simulink model "microNole_MPC2021"  (R2022b)
settings: Solver=VariableStepAuto  StartTime=0.0  StopTime=100  RelTol=1e-3
values from neighbouring files (symbols this model uses):
  Theta3 = Theta{1,3}    [MicroNole_dynamics.m]
  Theta4 = Theta{1,4}    [MicroNole_dynamics.m]
  Theta5 = Theta{1,5}    [MicroNole_dynamics.m]
  Theta6 = Theta3*Theta5/Theta4    [MicroNole_dynamics.m]
undefined symbols (not defined in the file or in its folder): b1, b2, b_bar, d0, desired_longitudinal_speed, double_lane_flag, F1, F2, h, H1, H2, H_bar, K1, K_mpc_clock, K_mpc_counterclock, Ki1, Kp1, L, M, n_input, n_states, omegam0, p1, p2, rg, Rw, sat_pwm, sat_steering, Theta1, Theta2, Ts, V0, X0, x_boundary
settings Model: Creator=zysgh  LastModifiedBy=Abelb
settings DebuggingCC: UnconnectedInputMsg=warning  UnconnectedOutputMsg=warning  UnconnectedLineMsg=warning
settings ModelReferenceCC: EnableRefExpFcnMdlSchedulingChecks=on
settings RTWCC: DLArmComputeVersion=19.05

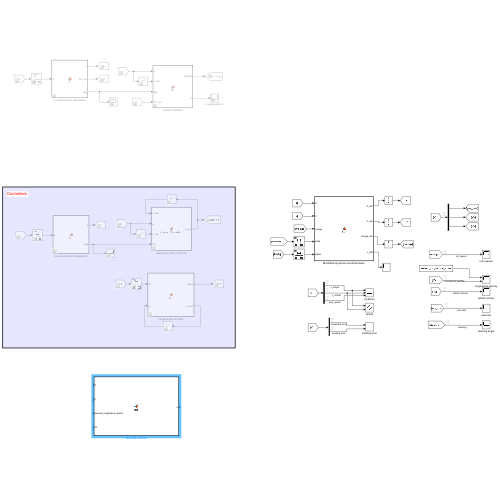
[thumbnail: Simulink's stored preview of the top-level diagram]
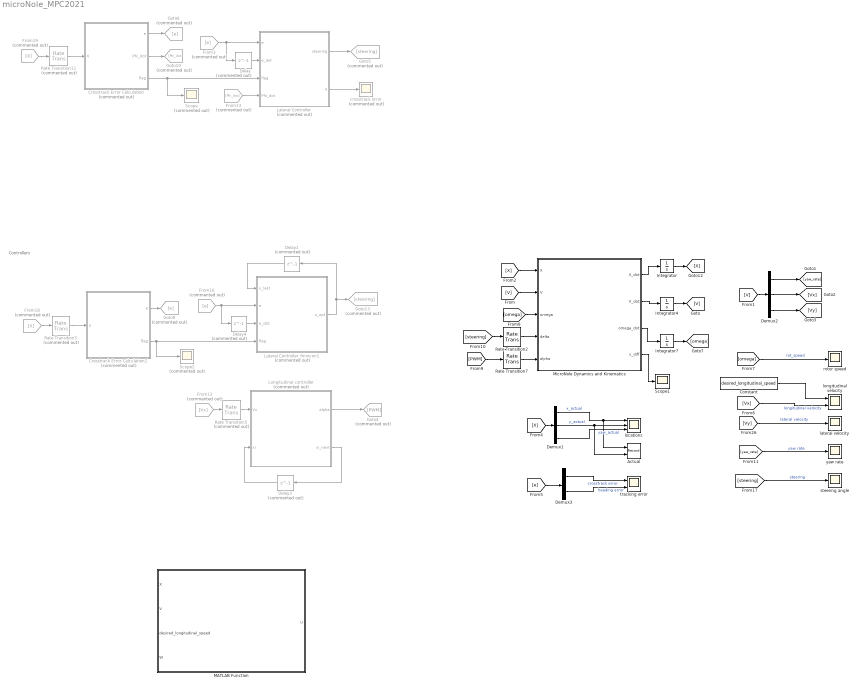
== system microNole_MPC2021 ==
  note: Controllers
  Actual : Record  FileSettingsInternal="{\"entries\":[{\"content\":{\"excelSettings\":{\"content\":{},\"type\":\"Streamout.ExcelSettings\"}},\"type\":\"Streamout.FileSettingStorage\",\"uuid\":\"74785e19-3353-448a-b1e4-8c9a9f0e60d2\"}],\"packageUris\":[\"http://schema.mathworks.com/mf0/streamout_blocks/R2020a\"],\"version\":\"1.0\"}"  Layout=[1 1]  SignalsInternal="{\"entries\":[{\"content\":{\"signals\":[{\"content\":{\"blockPath\":[\"microNole_MPC2021/Actual\"],\"channel\":[],\"dimensions\":[1],\"domain\":\"microNole_MPC2021/Actual\",\"lineColor\":\"#a2142f\",\"plots\":[1],\"port\":1,\"sid\":[\"\"],\"signalID\":1557,\"signalName\":\"x_actual\"},\"type\":\"RecordBlkView.Signal\",\"uuid\":\"f191aebf-62f9-445e-8cf5-1f0d9c420840\"},{\"content\":{\"blockPath\":[\"microNole_MPC2021/Actual\"],\"channel\":[],\"dimensions\":[1],\"domain\":\"microNole_MPC2021/Actual\",\"lineColor\":\"#139fff\",\"plots\":[1],\"port\":2,\"sid\":[\"\"],\"signalID\":1561,\"signalName\":\"y_actual\"},\"type\":\"RecordBlkView.Signal\",\"uuid\":\"59f82387-b242-4805-80ba-ae25613a261f\"}]},\"type\":\"RecordBlkView.InputSignals\",\"uuid\":\"e4cdd9aa-afbb-4b03-ab14-af52f1503f9a\"}],\"packageUris\":[\"http://schema.mathworks.com/mf0/streamout_blocks/R2020a\"],\"version\":\"1.0\"}"  VisualizationBindings="{\"xyplotplugin\":{\"info\":[{\"series\":[{\"bindingParametersList\":[{\"parameter\":\"X-Axis\",\"signalID\":1557,\"signalName\":\"x_actual\"},{\"parameter\":\"Y-Axis\",\"signalID\":1561,\"signalName\":\"y_actual\"}],\"seriesID\":12829}],\"subplotID\":1}]}}"  CompatibilityTag=XY  st=-1
  Constant : Constant  Value=desired_longitudinal_speed
  Crosstrack Error Calculation : MATLAB Function  Commented=on  TreatAsAtomicUnit=on
  Crosstrack Error Calculation2 : MATLAB Function  Commented=on  TreatAsAtomicUnit=on
  Delay : Delay  Commented=on  DelayLength=1  InitialCondition=[e10; e20]  SampleTime=Ts
  Delay1 : Delay  Commented=on  DelayLength=1  SampleTime=Ts
  Delay3 : Delay  Commented=on  DelayLength=1  SampleTime=Ts
  Delay4 : Delay  Commented=on  DelayLength=1  InitialCondition=[e10; e20]  SampleTime=Ts
  Demux1 : Demux  Outputs=3
  Demux2 : Demux  Outputs=3
  Demux3 : Demux  Outputs=2
  From12 : From  Commented=on  GotoTag=Vx
  From13 : From  Commented=on  GotoTag=Phi_dot
  From16 : From  Commented=on  GotoTag=e
  From18 : From  Commented=on  GotoTag=X
  From19 : From  Commented=on  GotoTag=X
  From3 : From  Commented=on  GotoTag=e
  Goto10 : Goto  Commented=on  GotoTag=Phi_dot
  Goto13 : Goto  Commented=on  GotoTag=steering
  Goto4 : Goto  Commented=on  GotoTag=PWM
  Goto5 : Goto  Commented=on  GotoTag=steering
  Goto6 : Goto  Commented=on  GotoTag=e
  Goto9 : Goto  Commented=on  GotoTag=e
  Integrator : Integrator  InitialCondition=X0
  Integrator4 : Integrator  InitialCondition=V0
  Integrator7 : Integrator  InitialCondition=omegam0
  Lateral Controller : MATLAB Function  Commented=on  TreatAsAtomicUnit=on
  Lateral Controller_fmincon1 : MATLAB Function  Commented=on  TreatAsAtomicUnit=on
  Longitudinal controller : MATLAB Function  Commented=on  TreatAsAtomicUnit=on
  MATLAB Function : MATLAB Function  TreatAsAtomicUnit=on
  MicroNole Dynamics and Kinematics : MATLAB Function  TreatAsAtomicUnit=on
  Rate Transition11 : RateTransition  Commented=on  InitialCondition=X0  OutPortSampleTime=Ts
  Rate Transition2 : RateTransition  Integrity=off  OutPortSampleTime=0
  Rate Transition3 : RateTransition  Commented=on  InitialCondition=X0  OutPortSampleTime=Ts
  Rate Transition5 : RateTransition  Commented=on  OutPortSampleTime=Ts
  Rate Transition7 : RateTransition  Integrity=off  OutPortSampleTime=0
  Scope : Scope  Commented=on
  Scope1 : Scope
  Scope2 : Scope  Commented=on
  crosstrack error : Scope  Commented=on
  lateral velocity : Scope
  locations : Scope  NumInputPorts=3
  longitudinal velocity : Scope  NumInputPorts=2
  rotor speed : Scope
  steering angle : Scope
  tracking error : Scope  NumInputPorts=2
  yaw rate : Scope
  wires:
  [X] -> Demux1/1
  Demux1/1 -> Actual/1, locations/1  "x_actual"
  Demux1/2 -> Actual/2, locations/2  "y_actual"
  Demux1/3 -> locations/3  "yaw_actual"
  MicroNole Dynamics and Kinematics/3(omega_dot) -> Integrator7/1
  [omega] -> rotor speed/1  "rot_speed"
  [Vy] -> lateral velocity/1  "lateral velocity"
  MicroNole Dynamics and Kinematics/2(V_dot) -> Integrator4/1
  [V] -> MicroNole Dynamics and Kinematics/2(V)
  [omega] -> MicroNole Dynamics and Kinematics/3(omega)
  Integrator7/1 -> [omega]
  Integrator4/1 -> [V]
  [V] -> Demux2/1
  Demux2/1 -> [yaw_rate]
  Demux2/2 -> [Vx]
  Demux2/3 -> [Vy]
  MicroNole Dynamics and Kinematics/1(X_dot) -> Integrator/1
  Integrator/1 -> [X]
  [X] -> MicroNole Dynamics and Kinematics/1(X)
  Delay3/1 -> Longitudinal controller/2(xi)
  From12/1 -> Rate Transition5/1
  Rate Transition5/1 -> Longitudinal controller/1(Vx)
  Longitudinal controller/2(xi_next) -> Delay3/1
  From19/1 -> Rate Transition11/1
  Lateral Controller/2(e) -> crosstrack error/1
  Lateral Controller/1(steering) -> Goto5/1
  Rate Transition11/1 -> Crosstrack Error Calculation/1(X)
  Crosstrack Error Calculation/1(e) -> Goto6/1
  [Vx] -> longitudinal velocity/2  "longitudinal velocity"
  [yaw_rate] -> yaw rate/1  "yaw rate"
  [e] -> Demux3/1
  Demux3/1 -> tracking error/1  "crosstrack error"
  Demux3/2 -> tracking error/2  "heading error"
  Constant/1 -> longitudinal velocity/1
  [steering] -> Rate Transition2/1
  Rate Transition2/1 -> MicroNole Dynamics and Kinematics/4(delta)
  Longitudinal controller/1(alpha) -> Goto4/1
  [PWM] -> Rate Transition7/1
  Rate Transition7/1 -> MicroNole Dynamics and Kinematics/5(alpha)
  Delay/1 -> Lateral Controller/2(e_dot)
  From3/1 -> Delay/1, Lateral Controller/1("e ")
  Crosstrack Error Calculation/2(Phi_dot) -> Goto10/1
  From13/1 -> Lateral Controller/4(Phi_dot)
  [steering] -> steering angle/1  "steering"
  Crosstrack Error Calculation/3(flag) -> Scope/1, Lateral Controller/3(flag)
  Crosstrack Error Calculation2/1(e) -> Goto9/1
  Crosstrack Error Calculation2/2(flag) -> Scope2/1, Lateral Controller_fmincon1/4(flag)
  From18/1 -> Rate Transition3/1
  Delay4/1 -> Lateral Controller_fmincon1/3(e_dot)
  Rate Transition3/1 -> Crosstrack Error Calculation2/1(X)
  From16/1 -> Delay4/1, Lateral Controller_fmincon1/2(e)
  Lateral Controller_fmincon1/1(u_opt) -> Delay1/1, Goto13/1
  Delay1/1 -> Lateral Controller_fmincon1/1(u_last)
  MicroNole Dynamics and Kinematics/4(v_diff) -> Scope1/1

== matlab function microNole_MPC2021/MATLAB Function ==
  data: X input; V input; u output; desired_longitudinal_speed input; W input
function u = fcn(X,V,desired_longitudinal_speed,W)


coder.extrinsic('MicroNole_dynamics');
coder.extrinsic('MicroNole_kinematics');

fmincon()

== matlab function microNole_MPC2021/Crosstrack Error Calculation2 ==
  data: X input; p1 parameter; e output; double_lane_flag parameter; flag output; x_boundary parameter; p2 parameter
function [e,flag] = fcn(X,p1,double_lane_flag, x_boundary, p2)
% for double trajectory: [e,Phi_dot,flag] = fcn(X,p1,p2, x_boundary,double_lane_flag)
% for single trajectory: [e,Phi_dot,flag] = fcn(X,p1,double_lane_flag)


%% crosstrack error calculation
x = X(1);
y = X(2);
omegaz = X(3);


% %%%%%%%%%%%% 2. polynomial  %%%%%%%%%%%%
p = p1;
if double_lane_flag == 1  % if there exists double trajectorys?
    if x <= x_boundary
        p = p1;
    else
        p = p2;
    end
end
[e1,e2,Phi_dot,flag] = crosstrack_error(x,y,p,omegaz);

e = [e1;
     e2];

== matlab function microNole_MPC2021/Lateral Controller_fmincon1 ==
  data: u_last input; e input; e_dot input; flag input; F1 parameter; F2 parameter; H_bar parameter; b_bar parameter; u_opt output; M parameter; n_states parameter; n_input parameter; h parameter; H1 parameter; H2 parameter; b1 parameter; b2 parameter
function u_opt  = Lateral_Controller1(u_last,e, e_dot, flag, F1,F2,H_bar,b_bar, M, n_states, n_input,h,H1,H2,b1,b2)

E = [e(1);e_dot(1);e(2);e_dot(2)];


coder.extrinsic('constrained_MPC_quaprog')
coder.extrinsic('constrained_MPC_pgdhb')
%% feedback term: constrained MPC-based controller
% online optimization
u_opt = zeros(n_input,1);
% u_opt(:) = constrained_MPC_quaprog(E,u_last,M,F1,H_bar,b_bar,h,n_states,n_input);
u_opt(:) = constrained_MPC_pgdhb(E,u_last,M,F1,H1,H2,b1,b2,h,n_states,n_input);
% 1: counter clockwise; -1: clockwise
if flag == -1
%     u_opt(:) = constrained_MPC_quaprog(E,u_last,M,F2,H_bar,b_bar,h,n_states,n_input);
    u_opt(:) = constrained_MPC_pgdhb(E,u_last,M,F2,H1,H2,b1,b2,h,n_states,n_input);
end
    
%% feedforward term
% the steady error on lateral distance could be vanished
% the steady error on heading error could not be vanished, it is because
% the slips angles at the rear and front wheels are completely determined.
% Vx = desired_longitudinal_speed;
% if Phi_dot == 0
%     delta_ff = 0;
% else
%     R = Vx/Phi_dot;
%     delta_ff = -K_mpc(3)*(Theta5-Vx)/(2*R*Theta6) + (L^2)*Vx*(Theta3+Theta4)/(2*R*b2) - b1*K_mpc(3)*(L^2)*(Theta3+Theta4)/(4*R*Theta6*b2);
% end

== matlab function microNole_MPC2021/Lateral Controller ==
  data: e input; e_dot input; K_mpc_clock parameter; b1 parameter; b2 parameter; flag input; Phi_dot input; Theta5 parameter; Theta6 parameter; Theta3 parameter; Theta4 parameter; L parameter; steering output; e output; desired_longitudinal_speed parameter; K_mpc_counterclock parameter
function [steering,e] = fcn(e, e_dot, K_mpc_clock,b1, b2,flag,Phi_dot, Theta5, Theta6, Theta3, Theta4, L,desired_longitudinal_speed, K_mpc_counterclock)

E = [e(1);e_dot(1);e(2);e_dot(2)];

%% controller
K_mpc = K_mpc_counterclock;
% 1: counter clockwise; -1: clockwise
if flag == -1
    K_mpc = K_mpc_clock;
end
    
% feedforward term
% the steady error on lateral distance could be vanished
% the steady error on heading error could not be vanished, it is because
% the slips angles at the rear and front wheels are completely determined.
Vx = desired_longitudinal_speed;
if Phi_dot == 0
    delta_ff = 0;
else
    R = Vx/Phi_dot;
    delta_ff = -K_mpc(3)*(Theta5-Vx)/(2*R*Theta6) + (L^2)*Vx*(Theta3+Theta4)/(2*R*b2) - b1*K_mpc(3)*(L^2)*(Theta3+Theta4)/(4*R*Theta6*b2);
end

% feeback
% steering = k_mpc * E + 2*sign(E)*d0;
steering = K_mpc * E + delta_ff;

== matlab function microNole_MPC2021/MicroNole Dynamics and Kinematics ==
  data: X input; X_dot output; V input; V_dot output; omega input; delta input; alpha input; omega_dot output; Theta2 parameter; Theta3 parameter; Theta4 parameter; L parameter; Rw parameter; rg parameter; Theta1 parameter; Theta5 parameter; sat_pwm parameter; sat_steering parameter; d0 parameter; v_diff output
function [X_dot, V_dot, omega_dot,v_diff] = fcn(X, V, omega, delta,alpha, Theta2, Theta3, Theta4, L, Rw, rg, Theta1, Theta5,sat_pwm, sat_steering,d0)
%%
% States:
%        - X: [x,y,heading] world frame
%        - V: [Vx, Vy, yaw rate] car frame
%        - yaw: car yaw angle
%        - omega: motor rotation speed
% Inputs: 
%        - delta: steering angle
%        - alpha: throttle command (PWM%)
% parameters:
%

% %% command satuation
% if abs(alpha) > sat_pwm
%     alpha =  sign(alpha) * sat_pwm;
% end
if abs(delta) > sat_steering
    delta =  sign(delta) * sat_steering;
end
%% upacking inputs
yaw_rate = V(1);
Vx = V(2);
Vy = V(3);
Phi = X(3);

%% dynamical model
Theta6 = Theta3*Theta5/Theta4;

omega_dot = -Theta1 * omega + Theta2 * alpha;

A1 = (L/2) * Theta3 * delta * cos(delta);
B1 = (L/2) * Theta3 *(1-cos(delta));
C1 = ((1/2) * Theta3 * (1+cos(delta)) + Theta4) * (1/2) * L^2;
D1 = (Rw*L/(2*rg)) * Theta4 * sin(delta);
yaw_rate_dot = -C1*yaw_rate + A1*Vx + B1*Vy + D1*omega;

A2 = 2 * Theta5 + Theta6 * delta * sin(delta);
B2 = Theta6 * sin(delta);
C2 = L*Theta6*sin(delta)/2;
D2 = Theta5*Rw*(1+cos(delta))/rg;
Vx_dot = -A2*Vx + B2*Vy + C2*yaw_rate + yaw_rate*Vy + D2*omega;

A3 = Theta6 * delta * cos(delta);
B3 = Theta6 * (1+cos(delta));
C3 = L*(Theta6*(1-cos(delta))-2*Theta5)/2;
D3 = Theta5 * Rw *sin(delta)/rg;
Vy_dot = -B3*Vy + A3*Vx + C3*yaw_rate - yaw_rate*Vx + D3*omega;

%% forward kinematics (bickycle)
% v = sqrt(Vx^2 + Vy^2);
beta = atan(tan(delta)/2);
v = Vx*cos(beta);

x_dot = v * cos(Phi + beta);
y_dot = v * sin(Phi + beta);
Phi_dot = v * cos(beta) * tan(delta) / L;
% Phi_dot = yaw_rate;

% %% crosstrack kinematics
% ePhi = Phi_ref - Phi;
% d_dot = d0 - ((L*yaw_rate/2) * cos(ePhi) - Vx * sin(ePhi));



%% packing outputs
V_dot = [yaw_rate_dot;
         Vx_dot;
         Vy_dot];
     
X_dot = [x_dot;
         y_dot;
         Phi_dot];

== matlab function microNole_MPC2021/Longitudinal controller ==
  data: Vx input; xi input; Kp1 parameter; Ki1 parameter; K1 parameter; alpha output; xi_next output; Ts parameter; desired_longitudinal_speed parameter
function [alpha,xi_next] = fcn(Vx, xi, Kp1, Ki1,K1, Ts, desired_longitudinal_speed)
%% function [alpha,delta] = fcn(eVx, eOmegaz)
% low_level controller (PID) for yaw rate and longitudinal velocity
% Inputs:
%        - eVx: longitudinal velocity error = Vx_desired - Vx
%        - eOmegaz: yaw rate error = Omegaz_desired - Omegaz
% Outputs:
%        - alpha: PWM
%        - delta: steering angle
%
% Yu Zheng, RasLab, 01/04/2022

%% longitudinal velocity controller (PI)
eVx = desired_longitudinal_speed - Vx;
tau1 = 1;
tau2 = 1;
xi_next =  tau1 * xi + tau2 * eVx*Ts ;
alpha = K1 * desired_longitudinal_speed + Kp1 * eVx + Ki1 * xi;

== matlab function microNole_MPC2021/Crosstrack Error Calculation ==
  data: X input; p1 parameter; e output; double_lane_flag parameter; Phi_dot output; flag output; x_boundary parameter; p2 parameter
function [e,Phi_dot,flag] = fcn(X,p1,double_lane_flag, x_boundary, p2)
% for double trajectory: [e,Phi_dot,flag] = fcn(X,p1,p2, x_boundary,double_lane_flag)
% for single trajectory: [e,Phi_dot,flag] = fcn(X,p1,double_lane_flag)


%% crosstrack error calculation
x = X(1);
y = X(2);
omegaz = X(3);


% %%%%%%%%%%%% 2. polynomial  %%%%%%%%%%%%
p = p1;
if double_lane_flag == 1  % if there exists double trajectorys?
    if x <= x_boundary
        p = p1;
    else
        p = p2;
    end
end
[e1,e2,Phi_dot,flag] = crosstrack_error(x,y,p,omegaz);

e = [e1;
     e2];
